simulink model "template_rotary_inverted_pendulum_2018a"  (R2020a)
settings: Solver=FixedStepDiscrete  StartTime=0.0  StopTime=inf  FixedStep=0.005  RelTol=1e-3
values from neighbouring files (symbols this model uses):
  A = zeros(n_states)    [RIP.m]
  B = zeros(n_states,n_inputs)    [RIP.m]
  C = zeros(n_outputs, n_states)    [RIP.m]
  D = zeros(n_outputs, n_inputs)    [RIP.m]
  Ki = K_d_Int(:,1)    [RIP.m]
  Ks = K_d_Int(:,2:end)    [RIP.m]
  Ts = 1/200    (= 0.005)    [RIP.m]
  wc = 2*2*pi    (= 12.5663706144)    [RIP.m]
undefined symbols (not defined in the file or in its folder): National_Instruments, PCI
libraries: sldrtlib x2, simulink x2, simulink_extras x2
settings Model: SimulationMode=external  ExtModeTrigDuration=200000  Creator=magudelo  LastModifiedBy=user
settings SolverCC: InsertRTBMode=Always
settings DataIOCC: LimitDataPoints=on  SaveFormat=Array  SignalLoggingSaveFormat=ModelDataLogs  ReturnWorkspaceOutputs=off
settings OptimizationCC: ExpressionDepthLimit=2147483647
settings DebuggingCC: UnderspecifiedInitializationDetection=Classic  MergeDetectMultiDrivingBlocksExec=none  SolverPrmCheckMsg=warning  FcnCallInpInsideContextMsg=warning  StateNameClashWarn=warning  SFUnexpectedBacktrackingDiag=warning  SFNoUnconditionalDefaultTransitionDiag=warning  SFExecutionAtInitializationDiag=none  ArithmeticOperatorsInVariantConditions=warning
settings ModelReferenceCC: PropagateSignalLabelsOutOfModel=off
settings SFSimCC: SimUseLocalCustomCode=off  CustomCodeUndefinedFunction=UseInterfaceOnly
settings RTWCC: Description=Simulink Desktop Real-Time  SystemTargetFile=sldrt.tlc  TemplateMakefile=sldrt.tmf  RTWUseLocalCustomCode=off  RTWCompilerOptimization=on
settings CodeAppCC: MaxIdLength=95  StateflowObjectComments=on
settings TargetCC: TargetPreCompLibLocation=C:\Program Files\MATLAB\R2018a\toolbox\sldrt\lib\win64
settings ConfigComp: CovMetricSettings=dw  CovHtmlReporting=on  CovSaveCumulativeToWorkspaceVar=on  CovSaveSingleToWorkspaceVar=on  CovExternalEMLEnable=off

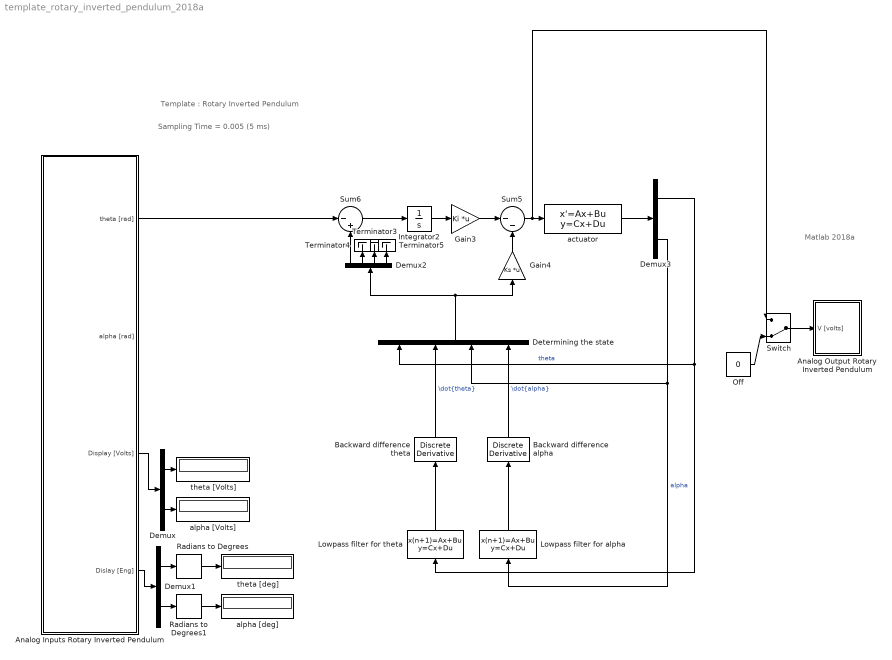
== system template_rotary_inverted_pendulum_2018a ==
  note: Matlab 2018a
  note: Sampling Time = 0.005 (5 ms)
  note: Template : Rotary Inverted Pendulum
  Analog Inputs Rotary Inverted Pendulum : Subsystem  mask(Analog Inputs. Rotary Inverted Pendulum){factor_theta=0.5959, offset_theta=-1.23, factor_alfa=0.3, offset_alfa=0.54}
      mask prompts: factor_theta "F_theta = Convertion factor from Volts to Radians (theta) :"; offset_theta "Off_theta = Offset for the angle of the arm (Volts):"; factor_alfa "F_alpha = Convertion Factor From Volts to Radians (alfa) :"; offset_alfa "Off_alpha = Offset for the angle of the rob (Volts) :"
      mask help:
      | Remember:
      |    Angle of the arm (theta) => channel ACH0
      |    Angle of the rod (alpha)    => channel ACH1
      |
      |   Angle of the arm  [rad] = F_theta * ( Angle of the arm [v]  + off_theta )
      |   Angle of the rod [rad] = F_alpha * ( Angle of the rod [v] + off_alpha )
  Analog Output Rotary Inverted Pendulum : Subsystem  mask(Analog Output - Rotary Inverted Pendulum){}
      mask help:
      | Remember
      |    AO 0 => Power Amplifier + Motor
  Backward difference alpha : simulink/Quick Insert/Discrete/Discrete Derivative  gainval=1.0  ICPrevScaledInput=0.0  OutMin=[]  OutMax=[]  OutDataType=fixdt(1, 16)  OutScaling=2^-10  DoSatur=off
      settings: SourceProductBaseCode=SL
  Backward difference theta : simulink/Quick Insert/Discrete/Discrete Derivative  gainval=1.0  ICPrevScaledInput=0.0  OutMin=[]  OutMax=[]  OutDataType=fixdt(1, 16)  OutScaling=2^-10  DoSatur=off
      settings: SourceProductBaseCode=SL
  Demux : Demux  Outputs=2
  Demux1 : Demux  Outputs=2
  Demux2 : Demux
  Demux3 : Demux  Outputs=2
  Determining the state : Mux
  Gain3 : Gain  Gain=Ki  Multiplication=Matrix(K*u)
  Gain4 : Gain  Gain=Ks  Multiplication=Matrix(K*u)
  Integrator2 : Integrator
  Lowpass filter for alpha : DiscreteStateSpace  A=1/(1 + wc*Ts)  B=wc*Ts/(1 + wc*Ts)  D=0  SampleTime=Ts
  Lowpass filter for theta : DiscreteStateSpace  A=1/(1 + wc*Ts)  B=wc*Ts/(1 + wc*Ts)  D=0  SampleTime=Ts
  Off : Constant  Value=0
  Radians to Degrees : simulink_extras/Transformations/Radians to Degrees
  Radians to Degrees1 : simulink_extras/Transformations/Radians to Degrees
  Sum5 : Sum  Inputs=|--
  Sum6 : Sum  Inputs=|-+
  "Switch  " : ManualSwitch  CurrentSetting=0
  Terminator3 : Terminator
  Terminator4 : Terminator
  Terminator5 : Terminator
  actuator : StateSpace  A=A  B=B  C=C  D=D  InitialCondition=0
  alpha [Volts] : Display
      settings: SampleTime=0.25
  alpha [deg] : Display
      settings: SampleTime=0.25
  theta [Volts] : Display
      settings: SampleTime=0.25
  theta [deg] : Display
      settings: SampleTime=0.25
  wires:
  Demux/1 -> theta [Volts]/1
  Demux/2 -> alpha [Volts]/1
  Analog Inputs Rotary Inverted Pendulum/3(Display [Volts]) -> Demux/1
  Analog Inputs Rotary Inverted Pendulum/4(Dislay [Eng]) -> Demux1/1
  Off/1 -> "Switch  "/2
  "Switch  "/1 -> Analog Output Rotary Inverted Pendulum/1(V [volts])
  Demux1/1 -> Radians to Degrees/1
  Radians to Degrees/1 -> theta [deg]/1
  Demux1/2 -> Radians to Degrees1/1
  Radians to Degrees1/1 -> alpha [deg]/1
  Analog Inputs Rotary Inverted Pendulum/1(theta [rad]) -> Sum6/1
  Gain3/1 -> Sum5/1
  Integrator2/1 -> Gain3/1
  Sum6/1 -> Integrator2/1
  Gain4/1 -> Sum5/2
  Demux2/4 -> Terminator5/1
  Determining the state/1 -> Gain4/1, Demux2/1
  Demux2/1 -> Sum6/2
  Demux2/2 -> Terminator4/1
  Demux2/3 -> Terminator3/1
  Lowpass filter for alpha/1 -> Backward difference alpha/1
  Backward difference alpha/1 -> Determining the state/4  "\\dot{alpha}"
  Lowpass filter for theta/1 -> Backward difference theta/1
  Backward difference theta/1 -> Determining the state/2  "\\dot{theta}"
  actuator/1 -> Demux3/1
  Sum5/1 -> "Switch  "/1, actuator/1
  Demux3/1 -> Determining the state/1, Lowpass filter for theta/1  "theta"
  Demux3/2 -> Determining the state/3, Lowpass filter for alpha/1  "alpha"

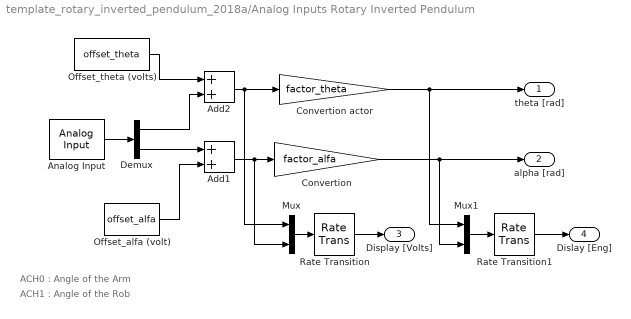
== system template_rotary_inverted_pendulum_2018a/Analog Inputs Rotary Inverted Pendulum ==
  note: ACH1 : Angle of the Rob
  note: ACH0 : Angle of the Arm
  Add1 : Sum
  Add2 : Sum
  Analog Input : sldrtlib/Analog Input  SampleTime=0.005  MaxMissedTicks=10  ShowMissedTicks=off  YieldWhenWaiting=off  DrvName=National_Instruments/PCI-6014  DrvAddress=4294967295  DrvOptions=[1 0 0 0 0 0]  Channels=[1 2]  RangeMode=1  VoltRange=1  DataType=1
      settings: AttributesFormatString=National Instruments\nPCI-6014 [auto]
  "Convertion " : Gain  Gain=factor_alfa
  Convertion actor : Gain  Gain=factor_theta
  Demux : Demux  Outputs=2
  Mux : Mux  Inputs=2
  Mux1 : Mux  Inputs=2
  Offset_alfa (volt) : Constant  Value=offset_alfa
  Offset_theta (volts) : Constant  Value=offset_theta
  Rate Transition : RateTransition  OutPortSampleTime=0.25
  Rate Transition1 : RateTransition  OutPortSampleTime=0.25
  theta [rad] : Outport  VectorParamsAs1DForOutWhenUnconnected=off
  alpha [rad] : Outport  Port=2  VectorParamsAs1DForOutWhenUnconnected=off
  Display [Volts] : Outport  Port=3  VectorParamsAs1DForOutWhenUnconnected=off
  Dislay [Eng] : Outport  Port=4  VectorParamsAs1DForOutWhenUnconnected=off
  wires:
  Rate Transition1/1 -> Dislay [Eng]/1
  Mux1/1 -> Rate Transition1/1
  Rate Transition/1 -> Display [Volts]/1
  Mux/1 -> Rate Transition/1
  "Convertion "/1 -> Mux1/2, alpha [rad]/1
  Add1/1 -> Mux/2, "Convertion "/1
  Offset_alfa (volt)/1 -> Add1/2
  Demux/2 -> Add1/1
  Convertion actor/1 -> Mux1/1, theta [rad]/1
  Offset_theta (volts)/1 -> Add2/1
  Add2/1 -> Mux/1, Convertion actor/1
  Demux/1 -> Add2/2
  Analog Input/1 -> Demux/1

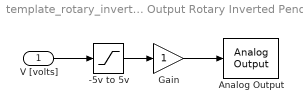
== system template_rotary_inverted_pendulum_2018a/Analog Output Rotary Inverted Pendulum ==
  V [volts] : Inport
  -5v to 5v : Saturate  UpperLimit=5  LowerLimit=-5
  Analog Output : sldrtlib/Analog Output  SampleTime=0.005  MaxMissedTicks=10  ShowMissedTicks=off  YieldWhenWaiting=off  DrvName=National_Instruments/PCI-6014  DrvAddress=4294967295  DrvOptions=[1 0 0 0 0 0]  Channels=1  RangeMode=1  VoltRange=1  InitialValue=0  FinalValue=0
      settings: AttributesFormatString=National Instruments\nPCI-6014 [auto]
  Gain : Gain
  wires:
  V [volts]/1 -> -5v to 5v/1
  -5v to 5v/1 -> Gain/1
  Gain/1 -> Analog Output/1
